simulink model "wlan_phy_tx_pmd"  (Simulink 7.8)
settings: Solver=VariableStepDiscrete  SolverMode=SingleTasking  StartTime=0.0  StopTime=inf  RelTol=1e-3
PostLoadFcn:
  | wlan_phy_tx_init
InitFcn:
  | wlan_phy_tx_init
StartFcn:
  | wlan_phy_tx_init
undefined symbols (not defined in the file): gcbh, ht_preamble_rom, MAX_CP_LEN, MAX_DATA_BITS_PER_SYM_PERIOD, MAX_NCBPS, MAX_NUM_BYTES, MAX_NUM_SC, MAX_NUM_SYMS, mcs_rom_11ag, mcs_rom_11n, Mod_Constellation_16QAM, Mod_Constellation_64QAM, Mod_Constellation_BPSK, Mod_Constellation_QPSK, Preamble_IQ, Preamble_IQ_scaled, tx_sim, wlan_tx_interleave_rom, xlBlockLoadCallback, xlGetNormalizedPeriod
libraries: xbsIndex_r4 x1358, xbsEDKLib_r4 x1
(part 5 of 10)

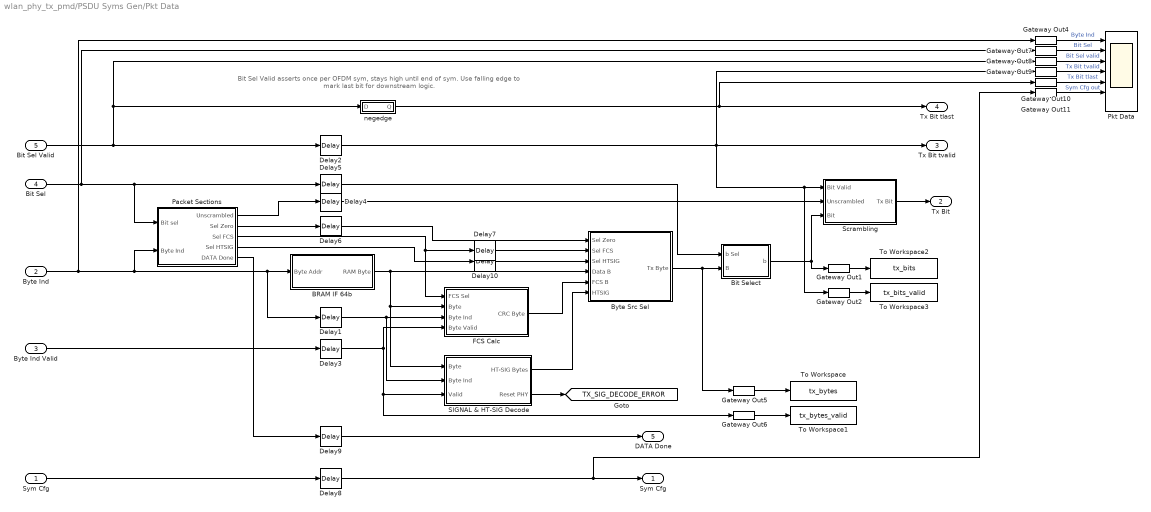
== system wlan_phy_tx_pmd/PSDU Syms Gen/Pkt Data ==
  note: Bit Sel Valid asserts once per OFDM sym,
      | stays high until end of sym. Use falling edge
      | to mark last bit for downstream logic.
  Sym Cfg : Inport
  Byte Ind : Inport  Port=2
  "Byte Ind Valid " : Inport  Port=3
  Bit Sel : Inport  Port=4
  Bit Sel Valid : Inport  Port=5
  BRAM IF 64b : Subsystem
  Bit Select : Subsystem
  Byte Src Sel : Subsystem
  Delay{1..10} (10 alike) : xbsIndex_r4/Delay  rst=off  infoeditControl=Selection of Reset will increase slice count due to use of real FFs and instead of SRLs  en=off  latency=1  dbl_ovrd=off  reg_retiming=off  block_type=delay
  FCS Calc : Subsystem
  Gateway Out{1..2,4..11} (10 alike) : xbsIndex_r4/Gateway Out  inherit_from_input=off  hdl_port=off  timing_constraint=None  locs_specified=off  LOCs={}  UseAsDAC=off  DACChannel='1'  block_type=gatewayout
  Packet Sections : Subsystem
  Pkt Data : Scope  NumInputPorts=7
      settings: YMin=-5~-5~-5~-5~-5~-5~-5  YMax=5~5~5~5~5~5~5  SaveName=ScopeData8
  SIGNAL & HT-SIG Decode : Subsystem
  Scrambling : Subsystem
  To Workspace : ToWorkspace  VariableName=tx_bytes  SampleTime=-1  SaveFormat=Array
  To Workspace1 : ToWorkspace  VariableName=tx_bytes_valid  SampleTime=-1  SaveFormat=Array
  To Workspace2 : ToWorkspace  VariableName=tx_bits  SampleTime=-1  SaveFormat=Array
  To Workspace3 : ToWorkspace  VariableName=tx_bits_valid  SampleTime=-1  SaveFormat=Array
  negedge : Subsystem
  " Sym Cfg" : Outport
  Tx Bit : Outport  Port=2
  Tx Bit tvalid : Outport  Port=3
  Tx Bit tlast : Outport  Port=4
  DATA Done : Outport  Port=5
  tag scope: TX_SIG_DECODE_ERROR=global
  wires:
  BRAM IF 64b/1(RAM Byte) -> Byte Src Sel/4(Data B), FCS Calc/2(Byte), SIGNAL & HT-SIG Decode/1(Byte)
  Delay3/1 -> FCS Calc/4(Byte Valid), SIGNAL & HT-SIG Decode/3(Valid), Gateway Out6/1
  FCS Calc/1(CRC Byte) -> Byte Src Sel/5(FCS B)
  Byte Src Sel/1(Tx Byte) -> Gateway Out5/1, Bit Select/2(B)
  Delay2/1 -> Tx Bit tvalid/1, Gateway Out9/1, Scrambling/1(Bit Valid), Gateway Out2/1
  "Byte Ind Valid "/1 -> Delay3/1
  Packet Sections/3(Sel FCS) -> FCS Calc/1(FCS Sel), Delay7/1
  Byte Ind/1 -> Packet Sections/2(Byte Ind), BRAM IF 64b/1(Byte Addr), Delay1/1, Gateway Out4/1
  Bit Sel/1 -> Delay5/1, Packet Sections/1(Bit sel), Gateway Out7/1
  Delay5/1 -> Bit Select/1(b Sel)
  Packet Sections/2(Sel Zero) -> Delay6/1
  Delay6/1 -> Byte Src Sel/1(Sel Zero)
  SIGNAL & HT-SIG Decode/2(Reset PHY) -> [TX_SIG_DECODE_ERROR]
  Bit Sel Valid/1 -> Delay2/1, negedge/1(D), Gateway Out8/1
  Bit Select/1(b) -> Scrambling/3(Bit), Gateway Out1/1
  Delay1/1 -> FCS Calc/3(Byte Ind), SIGNAL & HT-SIG Decode/2(Byte Ind)
  Packet Sections/1(Unscrambled) -> Delay4/1
  Delay4/1 -> Scrambling/2(Unscrambled)
  Scrambling/1(Tx Bit) -> Tx Bit/1
  Delay7/1 -> Byte Src Sel/2(Sel FCS)
  Sym Cfg/1 -> Delay8/1
  Delay8/1 -> " Sym Cfg"/1, Gateway Out11/1
  Packet Sections/5(DATA Done) -> Delay9/1
  Delay9/1 -> DATA Done/1
  negedge/1(Q) -> Tx Bit tlast/1, Gateway Out10/1
  Gateway Out5/1 -> To Workspace/1
  Gateway Out6/1 -> To Workspace1/1
  Gateway Out4/1 -> Pkt Data/1  "Byte Ind"
  Gateway Out7/1 -> Pkt Data/2  "Bit Sel"
  Gateway Out8/1 -> Pkt Data/3  "Bit Sel valid"
  Gateway Out9/1 -> Pkt Data/4  "Tx Bit tvalid"
  Gateway Out10/1 -> Pkt Data/5  "Tx Bit tlast"
  Gateway Out11/1 -> Pkt Data/6  "Sym Cfg out"
  SIGNAL & HT-SIG Decode/1(HT-SIG Bytes) -> Byte Src Sel/6(HTSIG)
  Packet Sections/4(Sel HTSIG) -> Delay10/1
  Gateway Out1/1 -> To Workspace2/1
  Gateway Out2/1 -> To Workspace3/1
  Delay10/1 -> Byte Src Sel/3("Sel HTSIG ")

== system wlan_phy_tx_pmd/PSDU Syms Gen/Puncture & Interleave ==
  note: Interleaver RAM stores all bits for one OFDM
      | symbol. Bits can be read immediately after last
      | bit for this OFDM sym is written to the RAM.
  Data Sym Ind : Inport
  Sym Cfg : Inport  Port=2
  Bit A : Inport  Port=3
  Bit B : Inport  Port=4
  Bits tvalid : Inport  Port=5
  Bits tlast : Inport  Port=6
  Delay{1..5} (5 alike) : xbsIndex_r4/Delay  rst=off  infoeditControl=Selection of Reset will increase slice count due to use of real FFs and instead of SRLs  en=off  latency=1  dbl_ovrd=off  reg_retiming=off  block_type=delay
  Delay6 : xbsIndex_r4/Delay  rst=off  infoeditControl=Selection of Reset will increase slice count due to use of real FFs and instead of SRLs  en=on  latency=1  dbl_ovrd=off  reg_retiming=off  block_type=delay
  Interleave RAM : Subsystem
  Interleaver Ctrl & Puncturing : Subsystem
  MCode : xbsIndex_r4/MCode  mfname=sym_config_decode  explicit_period=on  period=1  inputsTable={'boundInpExpr'=>[''],'inputs'=>['sym_cfg']}  outputsTable={'outputs'=>['load_base_rate','rotate_bpsk','load_htstf','load_htltf','load_full_rate','pilot_shift','cyclic_prefix','cyclic_shift'],'suppressOut'=>['off','off','off','off','off','off','off','off']}  dbl_ovrd=off  enable_stdout=off  enable_debug=off  suppress_output=on  defparams={}  hide_port_list={}  block_type=mcode
  Mem Sel : Subsystem
  " Sym Cfg" : Outport
  Sc Bits : Outport  Port=2
  Sym Bits Rdy : Outport  Port=3
  wires:
  Delay2/1 -> Interleave RAM/2(Bit B)
  Delay1/1 -> Interleave RAM/1(Bit A)
  Interleaver Ctrl & Puncturing/4(Wr B) -> Interleave RAM/6(Wr B), Delay6/2
  Interleaver Ctrl & Puncturing/3(Addr B) -> Interleave RAM/5(Bit Addr B)
  Interleaver Ctrl & Puncturing/2(Wr A) -> Interleave RAM/4(Wr A)
  Interleaver Ctrl & Puncturing/1(Addr A) -> Interleave RAM/3(Bit Addr A)
  MCode/1 -> Interleaver Ctrl & Puncturing/2(Base Rate)
  Bits tvalid/1 -> Interleaver Ctrl & Puncturing/1(Bits tvalid)
  Bit B/1 -> Delay2/1
  Bit A/1 -> Delay1/1
  Interleave RAM/1(Sc Bits) -> Sc Bits/1
  Data Sym Ind/1 -> Interleave RAM/7(Rd Addr)
  Delay3/1 -> Delay6/1
  Delay6/1 -> " Sym Cfg"/1
  Sym Cfg/1 -> Delay3/1, MCode/1
  Bits tlast/1 -> Delay4/1
  Delay4/1 -> Delay5/1, Mem Sel/1(En)
  Delay5/1 -> Sym Bits Rdy/1
  Mem Sel/1(Rd) -> Interleave RAM/8(Rd Mem Sel)
  Mem Sel/2(Wr) -> Interleave RAM/9(Wr Mem Sel)

== system wlan_phy_tx_pmd/Preamble & Outputs/DAC Outputs ==
  I : Inport
  Q : Inport  Port=2
  En : Inport  Port=3
  Ant Enables : Subsystem
  Inverter{1..4} (4 alike) : xbsIndex_r4/Inverter  en=off  latency=0  dbl_ovrd=off  block_type=inv
      settings: xl_area=[0 0 0 0 0 0 0]  block_version=VER_STRING_GOES_HERE
  Logical{,1..3} (4 alike) : xbsIndex_r4/Logical  logical_function=AND  inputs=2  en=off  latency=0  precision=Full  arith_type=Unsigned  n_bits=16  bin_pt=0  align_bp=on  dbl_ovrd=off  block_type=logical
  RFA DAC I : xbsIndex_r4/Gateway Out  inherit_from_input=off  hdl_port=on  timing_constraint=None  locs_specified=off  LOCs={}  UseAsDAC=off  DACChannel='1'  block_type=gatewayout
  RFA DAC Q : xbsIndex_r4/Gateway Out  inherit_from_input=off  hdl_port=on  timing_constraint=None  locs_specified=off  LOCs={}  UseAsDAC=off  DACChannel='1'  block_type=gatewayout
  RFB DAC I : xbsIndex_r4/Gateway Out  inherit_from_input=off  hdl_port=on  timing_constraint=None  locs_specified=off  LOCs={}  UseAsDAC=off  DACChannel='1'  block_type=gatewayout
  RFB DAC Q : xbsIndex_r4/Gateway Out  inherit_from_input=off  hdl_port=on  timing_constraint=None  locs_specified=off  LOCs={}  UseAsDAC=off  DACChannel='1'  block_type=gatewayout
  RFC DAC I : xbsIndex_r4/Gateway Out  inherit_from_input=off  hdl_port=on  timing_constraint=None  locs_specified=off  LOCs={}  UseAsDAC=off  DACChannel='1'  block_type=gatewayout
  RFC DAC Q : xbsIndex_r4/Gateway Out  inherit_from_input=off  hdl_port=on  timing_constraint=None  locs_specified=off  LOCs={}  UseAsDAC=off  DACChannel='1'  block_type=gatewayout
  RFD DAC I : xbsIndex_r4/Gateway Out  inherit_from_input=off  hdl_port=on  timing_constraint=None  locs_specified=off  LOCs={}  UseAsDAC=off  DACChannel='1'  block_type=gatewayout
  RFD DAC Q : xbsIndex_r4/Gateway Out  inherit_from_input=off  hdl_port=on  timing_constraint=None  locs_specified=off  LOCs={}  UseAsDAC=off  DACChannel='1'  block_type=gatewayout
  Register{,1..7} (8 alike) : xbsIndex_r4/Register  init=0  rst=on  en=off  dbl_ovrd=off  block_type=register
  Register10 : xbsIndex_r4/Register  init=0  rst=off  en=off  dbl_ovrd=off  block_type=register
  Register8 : xbsIndex_r4/Register  init=0  rst=off  en=off  dbl_ovrd=off  block_type=register
  Register9 : xbsIndex_r4/Register  init=0  rst=off  en=off  dbl_ovrd=off  block_type=register
  " I" : Outport
  " Q" : Outport  Port=2
  wires:
  Register1/1 -> RFA DAC Q/1
  Register/1 -> RFA DAC I/1
  Inverter1/1 -> Register/2, Register1/2
  Logical/1 -> Inverter1/1
  I/1 -> Register8/1
  RFA DAC I/1 -> " I"/1
  Q/1 -> Register10/1
  RFA DAC Q/1 -> " Q"/1
  Register3/1 -> RFB DAC Q/1
  Register2/1 -> RFB DAC I/1
  En/1 -> Register9/1
  Ant Enables/1(A En) -> Logical/2
  Logical1/1 -> Inverter2/1
  Inverter2/1 -> Register2/2, Register3/2
  Ant Enables/2(B En) -> Logical1/2
  Register5/1 -> RFC DAC Q/1
  Register4/1 -> RFC DAC I/1
  Logical2/1 -> Inverter3/1
  Inverter3/1 -> Register5/2, Register4/2
  Register7/1 -> RFD DAC Q/1
  Register6/1 -> RFD DAC I/1
  Logical3/1 -> Inverter4/1
  Inverter4/1 -> Register6/2, Register7/2
  Ant Enables/4(D En) -> Logical3/2
  Register8/1 -> Register/1, Register2/1, Register4/1, Register6/1
  Register9/1 -> Logical/1, Logical1/1, Logical2/1, Logical3/1
  Register10/1 -> Register1/1, Register3/1, Register5/1, Register7/1
  Ant Enables/3(C En) -> Logical2/2

== system wlan_phy_tx_pmd/Preamble & Outputs/End of Tx Ctrl ==
  note: Delay for latency between FIFO and
      | DAC outputs (scaling mults, output regs)
  FIFO Emtpy : Inport
  Tx Started : Inport  Port=2
  Delay2 : xbsIndex_r4/Delay  rst=off  infoeditControl=Selection of Reset will increase slice count due to use of real FFs and instead of SRLs  en=off  latency=4  dbl_ovrd=off  reg_retiming=off  block_type=delay
  Logical3 : xbsIndex_r4/Logical  logical_function=OR  inputs=2  en=off  latency=0  precision=Full  arith_type=Unsigned  n_bits=16  bin_pt=0  align_bp=on  dbl_ovrd=off  block_type=logical
  Posedge : Subsystem
  Posedge1 : Subsystem
  S-R Latch : Subsystem
  Output En : Outport
  wires:
  FIFO Emtpy/1 -> Posedge1/1(D)
  Tx Started/1 -> Posedge/1(D)
  Posedge/1(Q) -> S-R Latch/1(S)
  Logical3/1 -> S-R Latch/2(R)
  Delay2/1 -> Logical3/1
  Posedge1/1(Q) -> Delay2/1
  [TX_RESET] -> Logical3/2
  S-R Latch/1(Q) -> Output En/1

== system wlan_phy_tx_pmd/Preamble & Outputs/FIFO ==
  note: Use constant in place of actual FFT signal to debug timing
      | of samples at FIFO output and preamble/payload mux
  note: The register blocks around the FIFO fix apparent issues in hardware
      | where the FIFO would, on some downloads, insert an extra sample
      | after the preamble, before the payload. This is a sim/hardwrae mismatch
      | I never traced to a root cause. It definitely felt like a problem with
      | combinational signals driving the FIFO ports, somehow inducing
      | unexpected, seemingly asychronous, behaviors in hardware that do
      | not occur in simulation. The DFFs around the FIFO fixed it.
  Reset : Inport
  FFT I : Inport  Port=2
  FFT Q : Inport  Port=3
  Write : Inport  Port=4
  Rd : Inport  Port=5
  Constant2 : xbsIndex_r4/Constant  const=0  gui_display_data_type=Fixed-point  arith_type=Unsigned  n_bits=1  bin_pt=0  preci_type=Single  exp_width=8  frac_width=24  explicit_period=off  period=1  equ=P=C  opselect=C  inp2=PCIN>>17  opr=+  inp1=P  carry=CIN  dbl_ovrd=off  block_type=constant
  Constant3 : xbsIndex_r4/Constant  const=-1  gui_display_data_type=Fixed-point  arith_type=Signed (2's comp)  n_bits=16  bin_pt=15  preci_type=Single  exp_width=8  frac_width=24  explicit_period=on  period=1  equ=P=C  opselect=C  inp2=PCIN>>17  opr=+  inp1=P  carry=CIN  dbl_ovrd=off  block_type=constant
  Convert2 : xbsIndex_r4/Convert  gui_display_data_type=Boolean  arith_type=Boolean  n_bits=1  bin_pt=0  float_type=Single  exp_bits=8  fraction_bits=24  quantization=Truncate  overflow=Wrap  en=off  latency=0  dbl_ovrd=off  pipeline=off  block_type=convert
  Delay1 : xbsIndex_r4/Delay  rst=off  infoeditControl=Selection of Reset will increase slice count due to use of real FFs and instead of SRLs  en=off  latency=12  dbl_ovrd=off  reg_retiming=off  block_type=delay
  FIFO : xbsIndex_r4/FIFO  mem_type=Block RAM  performance_options=Standard_FIFO  infoedit1=Available only for V4, V5, V6, V7, K7, A7 and Zynq devices.  embedded_registers=on  depth=256  percent_nbits=1  rst=on  en=off  use_dcount=on  use_percent_full_port=off  use_almost_empty=off  almost_empty_thresh=2  use_almost_full=off  almost_full_thresh=14  dbl_ovrd=off  explicit_period=off  block_type=fifo
  I/Q Concat : Subsystem
  I/Q Slice : Subsystem
  Logical4 : xbsIndex_r4/Logical  logical_function=OR  inputs=2  en=off  latency=0  precision=Full  arith_type=Unsigned  n_bits=16  bin_pt=0  align_bp=on  dbl_ovrd=off  block_type=logical
  Register : xbsIndex_r4/Register  init=0  rst=off  en=off  dbl_ovrd=off  block_type=register
  Register1 : xbsIndex_r4/Register  init=0  rst=off  en=off  dbl_ovrd=off  block_type=register
  Register2 : xbsIndex_r4/Register  init=0  rst=off  en=off  dbl_ovrd=off  block_type=register
  Relational1 : xbsIndex_r4/Relational  mode=a=b  en=off  latency=0  dbl_ovrd=off  block_type=relational
  " I" : Outport
  " Q" : Outport  Port=2
  " Empty" : Outport  Port=3
  tag scope: OUTPUT_FIFO_OCC=global
  wires:
  FFT Q/1 -> I/Q Concat/2(Q)
  FFT I/1 -> I/Q Concat/1(I)
  I/Q Slice/2(Q) -> " Q"/1
  I/Q Slice/1(I) -> " I"/1
  I/Q Concat/1(IQ) -> Register/1
  Write/1 -> Register1/1
  [TX_RESET] -> Delay1/1
  FIFO/1 -> I/Q Slice/1(IQ)
  Rd/1 -> FIFO/3
  Delay1/1 -> Logical4/1
  Reset/1 -> Convert2/1
  Logical4/1 -> Register2/1
  Convert2/1 -> Logical4/2
  Register/1 -> FIFO/1
  Register1/1 -> FIFO/2
  Register2/1 -> FIFO/4
  FIFO/4 -> Relational1/1, [OUTPUT_FIFO_OCC]
  Constant2/1 -> Relational1/2
  Relational1/1 -> " Empty"/1

== system wlan_phy_tx_pmd/Preamble & Outputs/Posedge ==
  D : Inport
  Delay : xbsIndex_r4/Delay  rst=off  infoeditControl=Selection of Reset will increase slice count due to use of real FFs and instead of SRLs  en=off  latency=1  dbl_ovrd=off  reg_retiming=off  block_type=delay
      settings: infoedit=Hardware notes: A delay line is a chain, each link of which is an SRL16 followed by a flip-flop. If register retiming is enabled, the delay line is a chain of flip-flops.  xl_area=[1 1 0 0 0 0 0]  block_version=VER_STRING_GOES_HERE
  Inverter : xbsIndex_r4/Inverter  en=off  latency=0  dbl_ovrd=off  block_type=inv
      settings: xl_area=[0 0 0 0 0 0 0]  block_version=VER_STRING_GOES_HERE
  Logical1 : xbsIndex_r4/Logical  logical_function=AND  inputs=2  en=off  latency=0  precision=Full  arith_type=Unsigned  n_bits=8  bin_pt=2  align_bp=on  dbl_ovrd=off  block_type=logical
      settings: xl_area=[1 0 0 1 0 0 0]  block_version=VER_STRING_GOES_HERE
  Q : Outport
  wires:
  D/1 -> Logical1/2, Delay/1
  Logical1/1 -> Q/1
  Inverter/1 -> Logical1/1
  Delay/1 -> Inverter/1

== system wlan_phy_tx_pmd/Preamble & Outputs/Preamble Gen ==
  note: Synchronize preamble samples to the read_en signal
      | so the inputs to the mux are aligned
  note: TX_RESET asserts at the end of each Tx.
      | Delay it here to give the FIFO/MUX latencies
      | time to flush the last few samples before switching
      | the mux back to the preamble, for the next Tx.
  Tx Running : Inport
  Rd En : Inport  Port=2
  Constant3 : xbsIndex_r4/Constant  const=length(Preamble_IQ)-1  gui_display_data_type=Fixed-point  arith_type=Unsigned  n_bits=ceil(log2(length(Preamble_IQ)))  bin_pt=0  preci_type=Single  exp_width=8  frac_width=24  explicit_period=off  period=1  equ=P=C  opselect=C  inp2=PCIN>>17  opr=+  inp1=P  carry=CIN  dbl_ovrd=off  block_type=constant
  Counter : xbsIndex_r4/Counter  cnt_type=Free Running  cnt_to=Inf  operation=Up  start_count=0  cnt_by_val=1  arith_type=Unsigned  n_bits=ceil(log2(length(Preamble_IQ)))  bin_pt=0  load_pin=off  rst=on  en=on  explicit_period=off  period=1  dbl_ovrd=off  use_behavioral_HDL=off  implementation=Fabric  block_type=counter
  Delay4 : xbsIndex_r4/Delay  rst=off  infoeditControl=Selection of Reset will increase slice count due to use of real FFs and instead of SRLs  en=off  latency=4  dbl_ovrd=off  reg_retiming=off  block_type=delay
  Inverter1 : xbsIndex_r4/Inverter  en=off  latency=0  dbl_ovrd=off  block_type=inv
      settings: xl_area=[0 0 0 0 0 0 0]  block_version=VER_STRING_GOES_HERE
  Logical1 : xbsIndex_r4/Logical  logical_function=AND  inputs=3  en=off  latency=0  precision=Full  arith_type=Unsigned  n_bits=16  bin_pt=0  align_bp=on  dbl_ovrd=off  block_type=logical
  Preamble I : xbsIndex_r4/ROM  depth=length(Preamble_IQ_scaled)  initVector=real(Preamble_IQ_scaled)  distributed_mem=Distributed memory  rst=off  init_reg=0  en=off  latency=1  gui_display_data_type=Fixed-point  arith_type="Signed  (2's comp)"  n_bits=16  bin_pt=15  preci_type=Single  exp_width=8  frac_width=24  dbl_ovrd=off  optimize=Area  use_rpm=on  block_type=sprom
  Preamble Q : xbsIndex_r4/ROM  depth=length(Preamble_IQ_scaled)  initVector=imag(Preamble_IQ_scaled)  distributed_mem=Distributed memory  rst=off  init_reg=0  en=off  latency=1  gui_display_data_type=Fixed-point  arith_type="Signed  (2's comp)"  n_bits=16  bin_pt=15  preci_type=Single  exp_width=8  frac_width=24  dbl_ovrd=off  optimize=Area  use_rpm=on  block_type=sprom
  Register{,1..3} (4 alike) : xbsIndex_r4/Register  init=0  rst=on  en=on  dbl_ovrd=off  block_type=register
  Relational2 : xbsIndex_r4/Relational  mode=a<b  en=off  latency=0  dbl_ovrd=off  block_type=relational
  Done : Outport
  I : Outport  Port=2
  Q : Outport  Port=3
  Early Done : Outport  Port=4
  wires:
  Counter/1 -> Preamble I/1, Preamble Q/1, Relational2/1
  [TX_RESET] -> Delay4/1
  Logical1/1 -> Counter/2
  Relational2/1 -> Logical1/3, Inverter1/1
  Constant3/1 -> Relational2/2
  Tx Running/1 -> Logical1/1
  Rd En/1 -> Logical1/2, Register1/3, Register2/3, Register3/3, Register/3
  Preamble I/1 -> Register2/1
  Preamble Q/1 -> Register3/1
  Register/1 -> Early Done/1, Register1/1
  Delay4/1 -> Counter/1, Register/2, Register1/2, Register2/2, Register3/2
  Inverter1/1 -> Register/1
  Register1/1 -> Done/1
  Register2/1 -> I/1
  Register3/1 -> Q/1

== system wlan_phy_tx_pmd/Preamble & Outputs/S-R Latch ==
  S : Inport
  R : Inport  Port=2
  Constant1 : xbsIndex_r4/Constant  const=1  gui_display_data_type=Fixed-point  arith_type=Boolean  n_bits=1  bin_pt=0  preci_type=Single  exp_width=8  frac_width=24  explicit_period=off  period=1  equ=P=C  opselect=C  inp2=PCIN>>17  opr=+  inp1=P  carry=CIN  dbl_ovrd=off  block_type=constant
      settings: block_version=VER_STRING_GOES_HERE
  Convert1 : xbsIndex_r4/Convert  gui_display_data_type=Boolean  arith_type=Boolean  n_bits=1  bin_pt=0  float_type=Single  exp_bits=8  fraction_bits=24  quantization=Truncate  overflow=Wrap  en=off  latency=0  dbl_ovrd=off  pipeline=off  block_type=convert
  Convert2 : xbsIndex_r4/Convert  gui_display_data_type=Boolean  arith_type=Boolean  n_bits=1  bin_pt=0  float_type=Single  exp_bits=8  fraction_bits=24  quantization=Truncate  overflow=Wrap  en=off  latency=0  dbl_ovrd=off  pipeline=off  block_type=convert
  Register2 : xbsIndex_r4/Register  init=0  rst=on  en=on  dbl_ovrd=off  block_type=register
      settings: xl_area=[1 1 0 0 0 0 0]  block_version=VER_STRING_GOES_HERE
  Q : Outport
  wires:
  Convert2/1 -> Register2/3
  Convert1/1 -> Register2/2
  Constant1/1 -> Register2/1
  R/1 -> Convert1/1
  Register2/1 -> Q/1
  S/1 -> Convert2/1

== system wlan_phy_tx_pmd/Preamble & Outputs/Scaling ==
  Payload Sel : Inport
  Preamble I : Inport  Port=2
  Preamble Q : Inport  Port=3
  Payload I : Inport  Port=4
  Payload Q : Inport  Port=5
  Display : Display
  Display1 : Display
  Gateway Out1 : xbsIndex_r4/Gateway Out  inherit_from_input=off  hdl_port=off  timing_constraint=None  locs_specified=off  LOCs={}  UseAsDAC=off  DACChannel='1'  block_type=gatewayout
  Gateway Out5 : xbsIndex_r4/Gateway Out  inherit_from_input=off  hdl_port=off  timing_constraint=None  locs_specified=off  LOCs={}  UseAsDAC=off  DACChannel='1'  block_type=gatewayout
  Mult : xbsIndex_r4/Mult  precision=User Defined  arith_type="Signed  (2's comp)"  n_bits=12  bin_pt=11  quantization=Truncate  overflow=Saturate  en=off  latency=1  dbl_ovrd=off  use_behavioral_HDL=off  opt=Speed  use_embedded=on  optimum_pipeline=off  pipeline=on  use_rpm=on  placement_style=Triangular  block_type=mult
  Mult1 : xbsIndex_r4/Mult  precision=User Defined  arith_type="Signed  (2's comp)"  n_bits=12  bin_pt=11  quantization=Truncate  overflow=Saturate  en=off  latency=1  dbl_ovrd=off  use_behavioral_HDL=off  opt=Speed  use_embedded=on  optimum_pipeline=off  pipeline=on  use_rpm=on  placement_style=Triangular  block_type=mult
  Mux : xbsIndex_r4/Mux  inputs=2  en=off  latency=0  precision=Full  arith_type=Unsigned  n_bits=16  bin_pt=14  quantization=Truncate  overflow=Wrap  dbl_ovrd=off  block_type=mux
  Mux1 : xbsIndex_r4/Mux  inputs=2  en=off  latency=0  precision=Full  arith_type=Unsigned  n_bits=16  bin_pt=14  quantization=Truncate  overflow=Wrap  dbl_ovrd=off  block_type=mux
  Mux2 : xbsIndex_r4/Mux  inputs=2  en=off  latency=0  precision=Full  arith_type=Unsigned  n_bits=16  bin_pt=14  quantization=Truncate  overflow=Wrap  dbl_ovrd=off  block_type=mux
  Register1 : xbsIndex_r4/Register  init=0  rst=off  en=off  dbl_ovrd=off  block_type=register
  Register5 : xbsIndex_r4/Register  init=0  rst=off  en=off  dbl_ovrd=off  block_type=register
  Register8 : xbsIndex_r4/Register  init=0  rst=off  en=off  dbl_ovrd=off  block_type=register
  " I" : Outport
  " Q" : Outport  Port=2
  wires:
  Gateway Out1/1 -> Display1/1
  Gateway Out5/1 -> Display/1
  [regTx_Scaling_Preamble] -> Gateway Out1/1, Mux1/3
  Register5/1 -> Mux1/1
  [regTx_Scaling_Payload] -> Gateway Out5/1, Mux1/2
  Mux1/1 -> Mult1/1, Mult/2
  Register1/1 -> Mult1/2
  Register8/1 -> Mult/1
  Mult1/1 -> " Q"/1
  Mult/1 -> " I"/1
  Payload Sel/1 -> Register5/1, Mux/1, Mux2/1
  Mux/1 -> Register8/1
  Mux2/1 -> Register1/1
  Payload I/1 -> Mux/3
  Payload Q/1 -> Mux2/3
  Preamble I/1 -> Mux/2
  Preamble Q/1 -> Mux2/2

== system wlan_phy_tx_pmd/Registers/Status Bits ==
  Concat : xbsIndex_r4/Concat  num_inputs=2  dbl_ovrd=off  block_type=concat
  Constant : xbsIndex_r4/Constant  const=0  gui_display_data_type=Fixed-point  arith_type=Unsigned  n_bits=31  bin_pt=0  preci_type=Single  exp_width=8  frac_width=24  explicit_period=off  period=1  equ=P=C  opselect=C  inp2=PCIN>>17  opr=+  inp1=P  carry=CIN  dbl_ovrd=off  block_type=constant
  32b : Outport
  wires:
  [regTx_TX_RUNNING] -> Concat/2
  Constant/1 -> Concat/1
  Concat/1 -> 32b/1

== system wlan_phy_tx_pmd/Resets/Posedge1 ==
  note: Rising Edge Detection
  D : Inport
  Delay : xbsIndex_r4/Delay  rst=off  infoeditControl=Selection of Reset will increase slice count due to use of real FFs and instead of SRLs  en=off  latency=1  dbl_ovrd=off  reg_retiming=off  block_type=delay
      settings: infoedit=Hardware notes: A delay line is a chain, each link of which is an SRL16 followed by a flip-flop. If register retiming is enabled, the delay line is a chain of flip-flops.  xl_area=[1 1 0 0 0 0 0]  block_version=VER_STRING_GOES_HERE
  Inverter : xbsIndex_r4/Inverter  en=off  latency=0  dbl_ovrd=off  block_type=inv
      settings: xl_area=[0 0 0 0 0 0 0]  block_version=VER_STRING_GOES_HERE
  Logical1 : xbsIndex_r4/Logical  logical_function=AND  inputs=2  en=off  latency=0  precision=Full  arith_type=Unsigned  n_bits=8  bin_pt=2  align_bp=on  dbl_ovrd=off  block_type=logical
      settings: xl_area=[1 0 0 1 0 0 0]  block_version=VER_STRING_GOES_HERE
  Q : Outport
  wires:
  Delay/1 -> Inverter/1
  Inverter/1 -> Logical1/1
  Logical1/1 -> Q/1
  D/1 -> Delay/1, Logical1/2

== system wlan_phy_tx_pmd/Resets/S-R Latch ==
  S : Inport
  R : Inport  Port=2
  Constant1 : xbsIndex_r4/Constant  const=1  gui_display_data_type=Boolean  arith_type=Boolean  n_bits=1  bin_pt=0  preci_type=Single  exp_width=8  frac_width=24  explicit_period=off  period=1  equ=P=C  opselect=C  inp2=PCIN>>17  opr=+  inp1=P  carry=CIN  dbl_ovrd=off  block_type=constant
      settings: block_version=VER_STRING_GOES_HERE
  Convert1 : xbsIndex_r4/Convert  gui_display_data_type=Boolean  arith_type=Boolean  n_bits=1  bin_pt=0  float_type=Single  exp_bits=8  fraction_bits=24  quantization=Truncate  overflow=Wrap  en=off  latency=0  dbl_ovrd=off  pipeline=off  block_type=convert
  Convert2 : xbsIndex_r4/Convert  gui_display_data_type=Boolean  arith_type=Boolean  n_bits=1  bin_pt=0  float_type=Single  exp_bits=8  fraction_bits=24  quantization=Truncate  overflow=Wrap  en=off  latency=0  dbl_ovrd=off  pipeline=off  block_type=convert
  Register2 : xbsIndex_r4/Register  init=0  rst=on  en=on  dbl_ovrd=off  block_type=register
      settings: xl_area=[1 1 0 0 0 0 0]  block_version=VER_STRING_GOES_HERE
  Q : Outport
  wires:
  Convert2/1 -> Register2/3
  Convert1/1 -> Register2/2
  Constant1/1 -> Register2/1
  R/1 -> Convert1/1
  Register2/1 -> Q/1
  S/1 -> Convert2/1

== system wlan_phy_tx_pmd/Resets/Sim Reset ==
  Disregard Subsystem : xbsIndex_r4/Disregard Subsystem  Tag=discardX  block_type=disregard
  Sim Reset : xbsIndex_r4/Gateway In  gui_display_data_type=Boolean  arith_type=Boolean  n_bits=16  bin_pt=14  preci_type=Single  exp_width=8  frac_width=24  quantization="Round  (unbiased: +/- Inf)"  overflow=Saturate  period=1  dbl_ovrd=off  timing_constraint=None  locs_specified=off  LOCs={}  UseAsADC=off  ADCChannel='1'  inherit_from_input=off  hdl_port=on  block_type=gatewayin
  Step : Step  Time=10  Before=1  After=0  SampleTime=1
  Out1 : Outport
  wires:
  Step/1 -> Sim Reset/1
  Sim Reset/1 -> Out1/1

== system wlan_phy_tx_pmd/Start Ctrl/Add MAC Extension ==
  note: The 802.11 spec defines a 6 usec "extension" period that occurs
      | after the last sample is transmitted. The PHY does not transmit
      | anything during this extension. The extension is implemented by
      | delaying the "TX_DONE" output to the MAC.
  Tx Start : Inport
  IQ Done : Inport  Port=2
  Counter1 : xbsIndex_r4/Counter  cnt_type=Free Running  cnt_to=Inf  operation=Up  start_count=0  cnt_by_val=1  arith_type=Unsigned  n_bits=10  bin_pt=0  load_pin=off  rst=on  en=on  explicit_period=off  period=1  dbl_ovrd=off  use_behavioral_HDL=off  implementation=Fabric  block_type=counter
  Logical1 : xbsIndex_r4/Logical  logical_function=AND  inputs=2  en=off  latency=0  precision=Full  arith_type=Unsigned  n_bits=16  bin_pt=0  align_bp=on  dbl_ovrd=off  block_type=logical
  Logical2 : xbsIndex_r4/Logical  logical_function=OR  inputs=2  en=off  latency=0  precision=Full  arith_type=Unsigned  n_bits=16  bin_pt=0  align_bp=on  dbl_ovrd=off  block_type=logical
  Relational3 : xbsIndex_r4/Relational  mode=a>b  en=off  latency=0  dbl_ovrd=off  block_type=relational
  S-R Latch1 : Subsystem
  S-R Latch2 : Subsystem
  Tx Active : Outport
  wires:
  Relational3/1 -> Logical2/1
  [regTx_PostTx_Extension] -> Relational3/2
  Counter1/1 -> Relational3/1
  Logical2/1 -> Counter1/1, S-R Latch1/2(R), S-R Latch2/2(R)
  Logical1/1 -> Counter1/2
  [TX_FORCE_RESET] -> Logical2/2
  IQ Done/1 -> S-R Latch1/1(S)
  S-R Latch1/1(Q) -> Logical1/1
  [TX_IQ_SAMP_CE] -> Logical1/2
  Tx Start/1 -> S-R Latch2/1(S)
  S-R Latch2/1(Q) -> Tx Active/1

== system wlan_phy_tx_pmd/Start Ctrl/Add TXEN Extension ==
  note: Handle case of bad timing values (RxSig must
      | be later than RF Tx Dis; this OR handles case
      | of code getting this backwards)
  note: This block delays de-assertion of the radio's TXEN signal
      | for a software-programmed duration after the last sample
      | has been output to the DACs. This delay accounts for
      | the non-zero latency from the DAC input to the radio's
      | RF output. Without this delay the radio and amplifier
      | will be disabled too early, clipping the last few usec
      | of the transmitted waveform.
      |
      | The RxSig Valid output is used by the Rx PHY to unmask its
      | IQ inputs. This control path avoids any unintentional Rx
      | events during a Tx (i.e. due to RF coupling or transients
      | at the start of a Tx).
  IQ Done : Inport
  Counter1 : xbsIndex_r4/Counter  cnt_type=Free Running  cnt_to=Inf  operation=Up  start_count=0  cnt_by_val=1  arith_type=Unsigned  n_bits=10  bin_pt=0  load_pin=off  rst=on  en=on  explicit_period=off  period=1  dbl_ovrd=off  use_behavioral_HDL=off  implementation=Fabric  block_type=counter
  Display : Display
  Display1 : Display
  Gateway Out{1..6} (6 alike) : xbsIndex_r4/Gateway Out  inherit_from_input=off  hdl_port=off  timing_constraint=None  locs_specified=off  LOCs={}  UseAsDAC=off  DACChannel='1'  block_type=gatewayout
  Logical1 : xbsIndex_r4/Logical  logical_function=AND  inputs=2  en=off  latency=0  precision=Full  arith_type=Unsigned  n_bits=16  bin_pt=0  align_bp=on  dbl_ovrd=off  block_type=logical
  Logical2 : xbsIndex_r4/Logical  logical_function=OR  inputs=2  en=off  latency=0  precision=Full  arith_type=Unsigned  n_bits=16  bin_pt=0  align_bp=on  dbl_ovrd=off  block_type=logical
  Logical3 : xbsIndex_r4/Logical  logical_function=OR  inputs=2  en=off  latency=0  precision=Full  arith_type=Unsigned  n_bits=16  bin_pt=0  align_bp=on  dbl_ovrd=off  block_type=logical
  Posedge1 : Subsystem
  Posedge2 : Subsystem
  Posedge3 : Subsystem
  Relational1 : xbsIndex_r4/Relational  mode=a>b  en=off  latency=0  dbl_ovrd=off  block_type=relational
  Relational3 : xbsIndex_r4/Relational  mode=a>b  en=off  latency=0  dbl_ovrd=off  block_type=relational
  S-R Latch1 : Subsystem
  TxEn Extension : Scope  NumInputPorts=7
      settings: TimeRange=14000  YMin=0~0~-1~-1~-1~-1~-1  YMax=1~1~1~1~1~1~1  SaveName=ScopeData10
  RxSig Valid : Outport
  Disable RF Tx : Outport  Port=2
  wires:
  [TX_IQ_SAMP_CE] -> Logical1/2
  S-R Latch1/1(Q) -> Logical1/1, Gateway Out3/1
  IQ Done/1 -> Posedge1/1(D), Gateway Out2/1
  [TX_FORCE_RESET] -> Logical2/2
  Logical1/1 -> Counter1/2
  Logical2/1 -> S-R Latch1/2(R), Counter1/1
  Counter1/1 -> Relational3/1, Relational1/1, Gateway Out1/1
  [regTx_PostTx_RF_En_Extension] -> Relational3/2, Gateway Out5/1
  Posedge1/1(Q) -> S-R Latch1/1(S)
  [regTx_PostTx_RxSig_Valid] -> Relational1/2, Gateway Out6/1
  Relational3/1 -> Logical3/2
  Posedge2/1(Q) -> Disable RF Tx/1, Gateway Out4/1
  Relational1/1 -> Logical2/1, Posedge3/1(D), Logical3/1
  Posedge3/1(Q) -> RxSig Valid/1
  Logical3/1 -> Posedge2/1(D)
  Gateway Out2/1 -> TxEn Extension/1  "IQ Done"
  Gateway Out3/1 -> TxEn Extension/2  "IQ Done Latch"
  Gateway Out1/1 -> TxEn Extension/3  "Counter"
  Gateway Out4/1 -> TxEn Extension/4  "Disable RF Tx"
  Gateway Out5/1 -> Display/1
  Gateway Out6/1 -> Display1/1

== system wlan_phy_tx_pmd/Start Ctrl/PHY Mode Sel ==
  note: Select between software-configured and MAC-hardware-configured
      | PHY mode (11a/11n). The mode is captured only at the start
      | of each Tx. The register/input are ignored at all other times.
  Sw Tx : Inport
  Hw Tx : Inport  Port=2
  Convert : xbsIndex_r4/Convert  gui_display_data_type=Boolean  arith_type=Boolean  n_bits=16  bin_pt=14  float_type=Single  exp_bits=8  fraction_bits=24  quantization=Truncate  overflow=Wrap  en=off  latency=0  dbl_ovrd=off  pipeline=off  block_type=convert
  Convert1 : xbsIndex_r4/Convert  gui_display_data_type=Boolean  arith_type=Boolean  n_bits=16  bin_pt=14  float_type=Single  exp_bits=8  fraction_bits=24  quantization=Truncate  overflow=Wrap  en=off  latency=0  dbl_ovrd=off  pipeline=off  block_type=convert
  Logical1 : xbsIndex_r4/Logical  logical_function=OR  inputs=2  en=off  latency=0  precision=Full  arith_type=Unsigned  n_bits=16  bin_pt=0  align_bp=on  dbl_ovrd=off  block_type=logical
  Mux : xbsIndex_r4/Mux  inputs=2  en=off  latency=0  precision=Full  arith_type=Unsigned  n_bits=16  bin_pt=14  quantization=Truncate  overflow=Wrap  dbl_ovrd=off  block_type=mux
  Register1 : xbsIndex_r4/Register  init=0  rst=off  en=on  dbl_ovrd=off  block_type=register
      settings: xl_area=[1 1 0 0 0 0 0]  block_version=VER_STRING_GOES_HERE
  Register2 : xbsIndex_r4/Register  init=0  rst=off  en=on  dbl_ovrd=off  block_type=register
      settings: xl_area=[1 1 0 0 0 0 0]  block_version=VER_STRING_GOES_HERE
  Register3 : xbsIndex_r4/Register  init=0  rst=off  en=on  dbl_ovrd=off  block_type=register
      settings: xl_area=[1 1 0 0 0 0 0]  block_version=VER_STRING_GOES_HERE
  PHY Mode : Outport
  wires:
  Convert1/1 -> Register3/1, Logical1/2, Register2/2
  Convert/1 -> Logical1/1, Register1/2
  Logical1/1 -> Register3/2
  Hw Tx/1 -> Convert1/1
  Sw Tx/1 -> Convert/1
  Mux/1 -> PHY Mode/1
  Register3/1 -> Mux/1
  Register2/1 -> Mux/3
  Register1/1 -> Mux/2
  [regTx_SW_TX_PHY_MODE] -> Register1/1
  [MAC_IO_PHY_TX_PHY_MODE] -> Register2/1

== system wlan_phy_tx_pmd/Start Ctrl/Pkt Buf Sel ==
  note: Select between software-configured and MAC-hardware-configured
      | packet buffer index. The index is captured only at the start
      | of each Tx. The register/input are ignored at all other times.
  Sw Tx : Inport
  Hw Tx : Inport  Port=2
  Convert : xbsIndex_r4/Convert  gui_display_data_type=Boolean  arith_type=Boolean  n_bits=16  bin_pt=14  float_type=Single  exp_bits=8  fraction_bits=24  quantization=Truncate  overflow=Wrap  en=off  latency=0  dbl_ovrd=off  pipeline=off  block_type=convert
  Convert1 : xbsIndex_r4/Convert  gui_display_data_type=Boolean  arith_type=Boolean  n_bits=16  bin_pt=14  float_type=Single  exp_bits=8  fraction_bits=24  quantization=Truncate  overflow=Wrap  en=off  latency=0  dbl_ovrd=off  pipeline=off  block_type=convert
  Logical1 : xbsIndex_r4/Logical  logical_function=OR  inputs=2  en=off  latency=0  precision=Full  arith_type=Unsigned  n_bits=16  bin_pt=0  align_bp=on  dbl_ovrd=off  block_type=logical
  Mux : xbsIndex_r4/Mux  inputs=2  en=off  latency=0  precision=Full  arith_type=Unsigned  n_bits=16  bin_pt=14  quantization=Truncate  overflow=Wrap  dbl_ovrd=off  block_type=mux
  Register1 : xbsIndex_r4/Register  init=0  rst=off  en=on  dbl_ovrd=off  block_type=register
      settings: xl_area=[1 1 0 0 0 0 0]  block_version=VER_STRING_GOES_HERE
  Register2 : xbsIndex_r4/Register  init=0  rst=off  en=on  dbl_ovrd=off  block_type=register
      settings: xl_area=[1 1 0 0 0 0 0]  block_version=VER_STRING_GOES_HERE
  Register3 : xbsIndex_r4/Register  init=0  rst=off  en=on  dbl_ovrd=off  block_type=register
      settings: xl_area=[1 1 0 0 0 0 0]  block_version=VER_STRING_GOES_HERE
  Pkt Buf : Outport
  wires:
  [MAC_IO_PHY_TX_PKT_BUF] -> Register2/1
  [regTx_PKT_BUF_SEL] -> Register1/1
  Register1/1 -> Mux/2
  Register2/1 -> Mux/3
  Register3/1 -> Mux/1
  Mux/1 -> Pkt Buf/1
  Sw Tx/1 -> Convert/1
  Hw Tx/1 -> Convert1/1
  Logical1/1 -> Register3/2
  Convert/1 -> Register1/2, Logical1/1
  Convert1/1 -> Register2/2, Logical1/2, Register3/1

== system wlan_phy_tx_pmd/Start Ctrl/Posedge1 ==
  D : Inport
  Delay : xbsIndex_r4/Delay  rst=off  infoeditControl=Selection of Reset will increase slice count due to use of real FFs and instead of SRLs  en=off  latency=1  dbl_ovrd=off  reg_retiming=off  block_type=delay
      settings: infoedit=Hardware notes: A delay line is a chain, each link of which is an SRL16 followed by a flip-flop. If register retiming is enabled, the delay line is a chain of flip-flops.  xl_area=[1 1 0 0 0 0 0]  block_version=VER_STRING_GOES_HERE
  Inverter : xbsIndex_r4/Inverter  en=off  latency=0  dbl_ovrd=off  block_type=inv
      settings: xl_area=[0 0 0 0 0 0 0]  block_version=VER_STRING_GOES_HERE
  Logical1 : xbsIndex_r4/Logical  logical_function=AND  inputs=2  en=off  latency=0  precision=Full  arith_type=Unsigned  n_bits=8  bin_pt=2  align_bp=on  dbl_ovrd=off  block_type=logical
      settings: xl_area=[1 0 0 1 0 0 0]  block_version=VER_STRING_GOES_HERE
  Q : Outport
  wires:
  D/1 -> Logical1/2, Delay/1
  Logical1/1 -> Q/1
  Inverter/1 -> Logical1/1
  Delay/1 -> Inverter/1

== system wlan_phy_tx_pmd/Start Ctrl/Posedge2 ==
  D : Inport
  Delay : xbsIndex_r4/Delay  rst=off  infoeditControl=Selection of Reset will increase slice count due to use of real FFs and instead of SRLs  en=off  latency=1  dbl_ovrd=off  reg_retiming=off  block_type=delay
      settings: infoedit=Hardware notes: A delay line is a chain, each link of which is an SRL16 followed by a flip-flop. If register retiming is enabled, the delay line is a chain of flip-flops.  xl_area=[1 1 0 0 0 0 0]  block_version=VER_STRING_GOES_HERE
  Inverter : xbsIndex_r4/Inverter  en=off  latency=0  dbl_ovrd=off  block_type=inv
      settings: xl_area=[0 0 0 0 0 0 0]  block_version=VER_STRING_GOES_HERE
  Logical1 : xbsIndex_r4/Logical  logical_function=AND  inputs=2  en=off  latency=0  precision=Full  arith_type=Unsigned  n_bits=8  bin_pt=2  align_bp=on  dbl_ovrd=off  block_type=logical
      settings: xl_area=[1 0 0 1 0 0 0]  block_version=VER_STRING_GOES_HERE
  Q : Outport
  wires:
  Delay/1 -> Inverter/1
  Inverter/1 -> Logical1/1
  Logical1/1 -> Q/1
  D/1 -> Delay/1, Logical1/2

== system wlan_phy_tx_pmd/Start Ctrl/Posedge4 ==
  D : Inport
  Delay : xbsIndex_r4/Delay  rst=off  infoeditControl=Selection of Reset will increase slice count due to use of real FFs and instead of SRLs  en=off  latency=1  dbl_ovrd=off  reg_retiming=off  block_type=delay
      settings: infoedit=Hardware notes: A delay line is a chain, each link of which is an SRL16 followed by a flip-flop. If register retiming is enabled, the delay line is a chain of flip-flops.  xl_area=[1 1 0 0 0 0 0]  block_version=VER_STRING_GOES_HERE
  Inverter : xbsIndex_r4/Inverter  en=off  latency=0  dbl_ovrd=off  block_type=inv
      settings: xl_area=[0 0 0 0 0 0 0]  block_version=VER_STRING_GOES_HERE
  Logical1 : xbsIndex_r4/Logical  logical_function=AND  inputs=2  en=off  latency=0  precision=Full  arith_type=Unsigned  n_bits=8  bin_pt=2  align_bp=on  dbl_ovrd=off  block_type=logical
      settings: xl_area=[1 0 0 1 0 0 0]  block_version=VER_STRING_GOES_HERE
  Q : Outport
  wires:
  D/1 -> Logical1/2, Delay/1
  Logical1/1 -> Q/1
  Inverter/1 -> Logical1/1
  Delay/1 -> Inverter/1

== system wlan_phy_tx_pmd/Start Ctrl/Posedge5 ==
  D : Inport
  Delay : xbsIndex_r4/Delay  rst=off  infoeditControl=Selection of Reset will increase slice count due to use of real FFs and instead of SRLs  en=off  latency=1  dbl_ovrd=off  reg_retiming=off  block_type=delay
      settings: infoedit=Hardware notes: A delay line is a chain, each link of which is an SRL16 followed by a flip-flop. If register retiming is enabled, the delay line is a chain of flip-flops.  xl_area=[1 1 0 0 0 0 0]  block_version=VER_STRING_GOES_HERE
  Inverter : xbsIndex_r4/Inverter  en=off  latency=0  dbl_ovrd=off  block_type=inv
      settings: xl_area=[0 0 0 0 0 0 0]  block_version=VER_STRING_GOES_HERE
  Logical1 : xbsIndex_r4/Logical  logical_function=AND  inputs=2  en=off  latency=0  precision=Full  arith_type=Unsigned  n_bits=8  bin_pt=2  align_bp=on  dbl_ovrd=off  block_type=logical
      settings: xl_area=[1 0 0 1 0 0 0]  block_version=VER_STRING_GOES_HERE
  Q : Outport
  wires:
  Delay/1 -> Inverter/1
  Inverter/1 -> Logical1/1
  Logical1/1 -> Q/1
  D/1 -> Delay/1, Logical1/2

== system wlan_phy_tx_pmd/Start Ctrl/Radio TXEN/RXEN Control ==
  note: This logic handles the the transition betwen TX and RX modes in the
      | radio circuits. The delayed cross-connect between Tx and Rx ensures
      | the radio transitions through standby (TXEN=RXEN=0).
      |
      | The PHY generates a single RXEN signal. The software should configure
      | the radio_controller to use this RXEN signal for whichever RF interfaces
      | are required. The PHY generates 4 TXEN signals (one per interface),
      | allowing the Tx interface to be selected per packet by the MAC.
  Rx : Inport
  Tx : Inport  Port=2
  Convert1 : xbsIndex_r4/Convert  gui_display_data_type=Fixed-point  arith_type=Unsigned  n_bits=1  bin_pt=0  float_type=Single  exp_bits=8  fraction_bits=24  quantization=Truncate  overflow=Wrap  en=off  latency=0  dbl_ovrd=off  pipeline=off  block_type=convert
  Convert7 : xbsIndex_r4/Convert  gui_display_data_type=Fixed-point  arith_type=Unsigned  n_bits=1  bin_pt=0  float_type=Single  exp_bits=8  fraction_bits=24  quantization=Truncate  overflow=Wrap  en=off  latency=0  dbl_ovrd=off  pipeline=off  block_type=convert
  Convert8 : xbsIndex_r4/Convert  gui_display_data_type=Fixed-point  arith_type=Unsigned  n_bits=1  bin_pt=0  float_type=Single  exp_bits=8  fraction_bits=24  quantization=Truncate  overflow=Wrap  en=off  latency=0  dbl_ovrd=off  pipeline=off  block_type=convert
  Delay : xbsIndex_r4/Delay  rst=off  infoeditControl=Selection of Reset will increase slice count due to use of real FFs and instead of SRLs  en=off  latency=32  dbl_ovrd=off  reg_retiming=off  block_type=delay
  Delay1 : xbsIndex_r4/Delay  rst=off  infoeditControl=Selection of Reset will increase slice count due to use of real FFs and instead of SRLs  en=off  latency=32  dbl_ovrd=off  reg_retiming=off  block_type=delay
  Gateway Out2 : xbsIndex_r4/Gateway Out  inherit_from_input=off  hdl_port=off  timing_constraint=None  locs_specified=off  LOCs={}  UseAsDAC=off  DACChannel='1'  block_type=gatewayout
  Gateway Out3 : xbsIndex_r4/Gateway Out  inherit_from_input=off  hdl_port=off  timing_constraint=None  locs_specified=off  LOCs={}  UseAsDAC=off  DACChannel='1'  block_type=gatewayout
  Inverter : xbsIndex_r4/Inverter  en=off  latency=0  dbl_ovrd=off  block_type=inv
  Inverter2 : xbsIndex_r4/Inverter  en=off  latency=0  dbl_ovrd=off  block_type=inv
  Inverter3 : xbsIndex_r4/Inverter  en=off  latency=0  dbl_ovrd=off  block_type=inv
  Logical{1,4..6} (4 alike) : xbsIndex_r4/Logical  logical_function=OR  inputs=2  en=off  latency=0  precision=Full  arith_type=Unsigned  n_bits=16  bin_pt=0  align_bp=on  dbl_ovrd=off  block_type=logical
  Logical{3,7..10} (5 alike) : xbsIndex_r4/Logical  logical_function=AND  inputs=2  en=off  latency=0  precision=Full  arith_type=Unsigned  n_bits=16  bin_pt=0  align_bp=on  dbl_ovrd=off  block_type=logical
  Logical2 : xbsIndex_r4/Logical  logical_function=AND  inputs=3  en=off  latency=0  precision=Full  arith_type=Unsigned  n_bits=16  bin_pt=0  align_bp=on  dbl_ovrd=off  block_type=logical
  Radio TxEn-RxEn : Scope  NumInputPorts=7
      settings: TimeRange=14000  YMin=0~0~-1~-1~-1~-1~-1  YMax=1~1~1~1~1~1~1  SaveName=ScopeData6
  Register{1..5} (5 alike) : xbsIndex_r4/Register  init=0  rst=off  en=off  dbl_ovrd=off  block_type=register
  b0 : xbsIndex_r4/Slice  nbits=1  boolean_output=off  mode=Lower Bit Location + Width  bit1=0  base1=MSB of Input  bit0=0  base0=LSB of Input  dbl_ovrd=off  block_type=slice
  b1 : xbsIndex_r4/Slice  nbits=1  boolean_output=off  mode=Lower Bit Location + Width  bit1=0  base1=MSB of Input  bit0=1  base0=LSB of Input  dbl_ovrd=off  block_type=slice
  b2 : xbsIndex_r4/Slice  nbits=1  boolean_output=off  mode=Lower Bit Location + Width  bit1=0  base1=MSB of Input  bit0=2  base0=LSB of Input  dbl_ovrd=off  block_type=slice
  b3 : xbsIndex_r4/Slice  nbits=1  boolean_output=off  mode=Lower Bit Location + Width  bit1=0  base1=MSB of Input  bit0=3  base0=LSB of Input  dbl_ovrd=off  block_type=slice
  tag scope: RC_IO_RXEN=global, RC_IO_TXEN_A=global, RC_IO_TXEN_B=global, RC_IO_TXEN_C=global, RC_IO_TXEN_D=global
  wires:
  Logical2/1 -> Delay/1, Convert7/1
  Inverter2/1 -> Logical3/1
  Delay/1 -> Inverter2/1
  Delay1/1 -> Inverter3/1
  Inverter3/1 -> Logical2/3
  Logical3/1 -> Delay1/1, Convert8/1
  Convert7/1 -> Register4/1
  Register4/1 -> [RC_IO_RXEN], Gateway Out2/1  "RC_RXEN"
  Convert8/1 -> Logical10/1, Logical7/1, Logical8/1, Logical9/1
  [regTx_RC_RXEN_ENABLE] -> Logical2/1
  Rx/1 -> Logical2/2
  Tx/1 -> Logical3/2
  [regTx_Use_MAC_Ant_Masks] -> Inverter/1
  Register5/1 -> [RC_IO_TXEN_A], Gateway Out3/1
  [MAC_Tx_Ant_Mask] -> b0/1, b1/1, b2/1, b3/1
  b0/1 -> Logical4/2
  Inverter/1 -> Convert1/1
  b1/1 -> Logical1/2
  b2/1 -> Logical5/2
  b3/1 -> Logical6/2
  Logical4/1 -> Logical10/2
  Logical1/1 -> Logical7/2
  Logical5/1 -> Logical8/2
  Logical6/1 -> Logical9/2
  Logical10/1 -> Register5/1
  Register1/1 -> [RC_IO_TXEN_B]
  Register2/1 -> [RC_IO_TXEN_C]
  Register3/1 -> [RC_IO_TXEN_D]
  Logical7/1 -> Register1/1
  Logical8/1 -> Register2/1
  Logical9/1 -> Register3/1
  Convert1/1 -> Logical4/1, Logical1/1, Logical5/1, Logical6/1
  Gateway Out2/1 -> Radio TxEn-RxEn/1  "RC_RXEN"
  Gateway Out3/1 -> Radio TxEn-RxEn/2  "RC_TXEN_A"

== system wlan_phy_tx_pmd/Start Ctrl/S-R Latch ==
  S : Inport
  R : Inport  Port=2
  Constant1 : xbsIndex_r4/Constant  const=1  gui_display_data_type=Boolean  arith_type=Boolean  n_bits=1  bin_pt=0  preci_type=Single  exp_width=8  frac_width=24  explicit_period=off  period=1  equ=P=C  opselect=C  inp2=PCIN>>17  opr=+  inp1=P  carry=CIN  dbl_ovrd=off  block_type=constant
      settings: block_version=VER_STRING_GOES_HERE
  Convert1 : xbsIndex_r4/Convert  gui_display_data_type=Boolean  arith_type=Boolean  n_bits=1  bin_pt=0  float_type=Single  exp_bits=8  fraction_bits=24  quantization=Truncate  overflow=Wrap  en=off  latency=0  dbl_ovrd=off  pipeline=off  block_type=convert
  Convert2 : xbsIndex_r4/Convert  gui_display_data_type=Boolean  arith_type=Boolean  n_bits=1  bin_pt=0  float_type=Single  exp_bits=8  fraction_bits=24  quantization=Truncate  overflow=Wrap  en=off  latency=0  dbl_ovrd=off  pipeline=off  block_type=convert
  Register2 : xbsIndex_r4/Register  init=0  rst=on  en=on  dbl_ovrd=off  block_type=register
      settings: xl_area=[1 1 0 0 0 0 0]  block_version=VER_STRING_GOES_HERE
  Q : Outport
  wires:
  Convert2/1 -> Register2/3
  Convert1/1 -> Register2/2
  Constant1/1 -> Register2/1
  R/1 -> Convert1/1
  Register2/1 -> Q/1
  S/1 -> Convert2/1

== system wlan_phy_tx_pmd/Start Ctrl/S-R Latch1 ==
  S : Inport
  R : Inport  Port=2
  Constant1 : xbsIndex_r4/Constant  const=1  gui_display_data_type=Boolean  arith_type=Boolean  n_bits=1  bin_pt=0  preci_type=Single  exp_width=8  frac_width=24  explicit_period=off  period=1  equ=P=C  opselect=C  inp2=PCIN>>17  opr=+  inp1=P  carry=CIN  dbl_ovrd=off  block_type=constant
      settings: block_version=VER_STRING_GOES_HERE
  Convert1 : xbsIndex_r4/Convert  gui_display_data_type=Boolean  arith_type=Boolean  n_bits=1  bin_pt=0  float_type=Single  exp_bits=8  fraction_bits=24  quantization=Truncate  overflow=Wrap  en=off  latency=0  dbl_ovrd=off  pipeline=off  block_type=convert
  Convert2 : xbsIndex_r4/Convert  gui_display_data_type=Boolean  arith_type=Boolean  n_bits=1  bin_pt=0  float_type=Single  exp_bits=8  fraction_bits=24  quantization=Truncate  overflow=Wrap  en=off  latency=0  dbl_ovrd=off  pipeline=off  block_type=convert
  Register2 : xbsIndex_r4/Register  init=0  rst=on  en=on  dbl_ovrd=off  block_type=register
      settings: xl_area=[1 1 0 0 0 0 0]  block_version=VER_STRING_GOES_HERE
  Q : Outport
  wires:
  S/1 -> Convert2/1
  Register2/1 -> Q/1
  R/1 -> Convert1/1
  Constant1/1 -> Register2/1
  Convert1/1 -> Register2/2
  Convert2/1 -> Register2/3

== system wlan_phy_tx_pmd/Start Ctrl/S-R Latch2 ==
  S : Inport
  R : Inport  Port=2
  Constant1 : xbsIndex_r4/Constant  const=1  gui_display_data_type=Fixed-point  arith_type=Unsigned  n_bits=1  bin_pt=0  preci_type=Single  exp_width=8  frac_width=24  explicit_period=off  period=1  equ=P=C  opselect=C  inp2=PCIN>>17  opr=+  inp1=P  carry=CIN  dbl_ovrd=off  block_type=constant
      settings: block_version=VER_STRING_GOES_HERE
  Convert1 : xbsIndex_r4/Convert  gui_display_data_type=Boolean  arith_type=Boolean  n_bits=1  bin_pt=0  float_type=Single  exp_bits=8  fraction_bits=24  quantization=Truncate  overflow=Wrap  en=off  latency=0  dbl_ovrd=off  pipeline=off  block_type=convert
  Convert2 : xbsIndex_r4/Convert  gui_display_data_type=Boolean  arith_type=Boolean  n_bits=1  bin_pt=0  float_type=Single  exp_bits=8  fraction_bits=24  quantization=Truncate  overflow=Wrap  en=off  latency=0  dbl_ovrd=off  pipeline=off  block_type=convert
  Register2 : xbsIndex_r4/Register  init=0  rst=on  en=on  dbl_ovrd=off  block_type=register
      settings: xl_area=[1 1 0 0 0 0 0]  block_version=VER_STRING_GOES_HERE
  Q : Outport
  wires:
  S/1 -> Convert2/1
  Register2/1 -> Q/1
  R/1 -> Convert1/1
  Constant1/1 -> Register2/1
  Convert1/1 -> Register2/2
  Convert2/1 -> Register2/3
